simulink model "NE_zad2"  (R2022b)
settings: Solver=ode4  StartTime=0.0  StopTime=1.5  FixedStep=6e-4  RelTol=1e-3
values from neighbouring files (symbols this model uses):
  fie = (UN-IN*Rt)/(wN)    (= 2.67908610996)    [NE_proj_zad2.m]
  IN = 130.7    [NE_proj_zad1_script.m]    (also in NE_proj_zad2.m)
  J = (Js+0*Js)    (= 0.97)    [NE_proj_zad2.m]
  Kp = 1.5*UN/10    (= 66)    [NE_proj_zad1_script.m]    (also in NE_proj_zad2.m)
  KT = 10/(1.2*wN)    (= 0.0548810148593)    [NE_proj_zad1_script.m]    (also in NE_proj_zad2.m)
  Kw = J/(2*KT*kz*beta*fie)    [NE_proj_zad2.m]
  lambdaN = 1.8    [NE_proj_zad1_script.m]    (also in NE_proj_zad2.m)
  m = T1    [NE_proj_zad2.m]
  PN = 54e3    (= 54000)    [NE_proj_zad1_script.m]    (also in NE_proj_zad2.m)
  Rt = 0.254    [NE_proj_zad1_script.m]    (also in NE_proj_zad2.m)
  T = 0.001*Lt/Rt    (= 0.00641732283465)    [NE_proj_zad1_script.m]    (also in NE_proj_zad2.m)
  TR = 4*beta    (= 0.144)    [NE_proj_zad2.m]
  UN = 440    [NE_proj_zad1_script.m]    (also in NE_proj_zad2.m)
  uz0 = lambdaN*IN*(Y*B1)/(B1-beta)    [NE_proj_zad2.m]
  V = beta*(Y*Kp*B)/((B1-beta)*Rt)    [NE_proj_zad2.m]
  wN = nN*pi/30    (= 151.843644924)    [NE_proj_zad1_script.m]    (also in NE_proj_zad2.m)
  Y = 10/(2.5*IN)    (= 0.0306044376435)    [NE_proj_zad1_script.m]    (also in NE_proj_zad2.m = 0.0153022188217)
settings Model: Creator=womru  LastModifiedBy=womru
settings DataIOCC: SaveFormat=StructureWithTime  ReturnWorkspaceOutputs=off
settings OptimizationCC: ReuseModelBlockBuffer=on

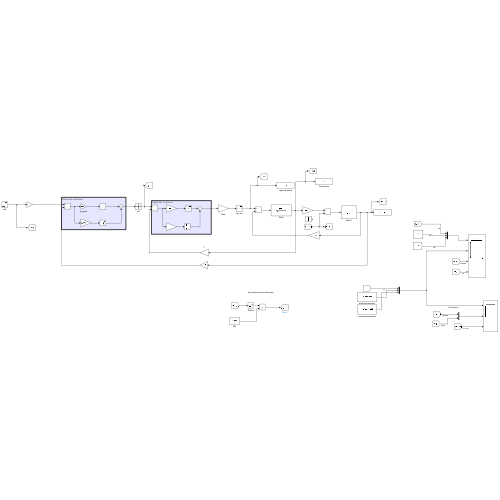
[thumbnail: Simulink's stored preview of the top-level diagram]
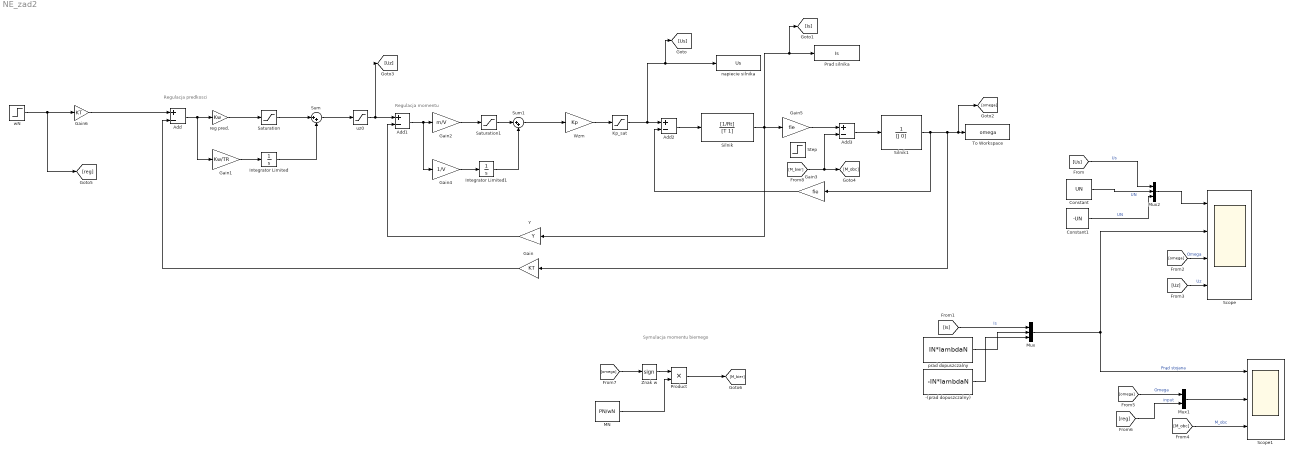
== system NE_zad2 ==
  note: Symulacja momentu biernego
  note: Regulacja momentu
  note: Regulacja predkosci
  -(prad dopuszczalny) : Constant  Value=-IN*lambdaN
  Add{,1..3} (4 alike) : Sum  Inputs=+-
  Constant : Constant  Value=UN
  Constant1 : Constant  Value=-UN
  Gain : Gain  Gain=KT
  Gain1 : Gain  Gain=Kw/TR
  Gain2 : Gain  Gain=m/V
  Gain3 : Gain  Gain=fie
  Gain4 : Gain  Gain=1/V
  Gain5 : Gain  Gain=fie
  Gain6 : Gain  Gain=KT
  Integrator Limited : Integrator  LimitOutput=on  UpperSaturationLimit=10  LowerSaturationLimit=-10
  Integrator Limited1 : Integrator  LimitOutput=on  UpperSaturationLimit=10  LowerSaturationLimit=-10
  Kp_sat : Saturate  UpperLimit=1.5*UN  LowerLimit=-1.5*UN
  MN : Constant  Value=PN/wN
  Mux : Mux  Inputs=3
  Mux1 : Mux  Inputs=2
  Mux2 : Mux  Inputs=3
  Prad silnika : ToWorkspace  VariableName=Is  SaveFormat=Structure With Time  SampleTime=-1
  Product : Product
  Saturation : Saturate  UpperLimit=10  LowerLimit=-10
  Saturation1 : Saturate  UpperLimit=10  LowerLimit=-10
  Scope : Scope  NumInputPorts=4
  Scope1 : Scope  NumInputPorts=3
  Silnik : TransferFcn  Numerator=[1/Rt]  Denominator=[T 1]
  Silnik1 : TransferFcn  Denominator=[J 0]
  Step : Step  Time=0  After=PN/wN  SampleTime=0
  Sum : Sum  Inputs=|++
  Sum1 : Sum  Inputs=|++
  To Workspace : ToWorkspace  VariableName=omega  SaveFormat=Structure With Time  SampleTime=-1
  Wzm : Gain  Gain=Kp
  Y : Gain  Gain=Y
  Znak w : Signum
  napiecie silnika : ToWorkspace  VariableName=Us  SaveFormat=Structure With Time  SampleTime=-1
  prad dopuszczalny : Constant  Value=IN*lambdaN
  reg pred. : Gain  Gain=Kw
  uz0 : Saturate  UpperLimit=abs(uz0)  LowerLimit=-1*abs(uz0)
  wN : Step  Time=0  After=wN  SampleTime=0
  wires:
  Add/1 -> Gain1/1, reg pred./1
  reg pred./1 -> Saturation/1
  Saturation/1 -> Sum/1
  Gain1/1 -> Integrator Limited/1
  Integrator Limited/1 -> Sum/2
  Sum/1 -> uz0/1
  uz0/1 -> [Uz], Add1/1
  Add1/1 -> Gain4/1, Gain2/1
  Gain2/1 -> Saturation1/1
  Saturation1/1 -> Sum1/1
  Sum1/1 -> Wzm/1
  Wzm/1 -> Kp_sat/1
  Gain4/1 -> Integrator Limited1/1
  Integrator Limited1/1 -> Sum1/2
  Add2/1 -> Silnik/1
  Gain5/1 -> Add3/1
  Add3/1 -> Silnik1/1
  Silnik1/1 -> Gain3/1, Gain/1, [omega], To Workspace/1
  Gain3/1 -> Add2/2
  Silnik/1 -> [Is], Prad silnika/1, Y/1, Gain5/1
  Y/1 -> Add1/2
  Gain/1 -> Add/2
  prad dopuszczalny/1 -> Mux/2
  Kp_sat/1 -> [Us], napiecie silnika/1, Add2/1
  [Us] -> Mux2/1  "Us"
  [Is] -> Mux/1  "Is"
  Mux/1 -> Scope1/1, Scope/2  "Prąd stojana"
  [omega] -> Scope/3  "Omega"
  [Uz] -> Scope/4  "Uz"
  Gain6/1 -> Add/1
  [M_obc] -> Scope1/3  "M_obc"
  Mux1/1 -> Scope1/2
  [omega] -> Mux1/1  "Omega"
  [reg] -> Mux1/2  "input"
  -(prad dopuszczalny)/1 -> Mux/3
  wN/1 -> [reg], Gain6/1
  [omega] -> Znak w/1
  Znak w/1 -> Product/1
  Product/1 -> [M_bier]
  MN/1 -> Product/2
  Mux2/1 -> Scope/1
  Constant/1 -> Mux2/2  "UN"
  Constant1/1 -> Mux2/3  "UN"
  [M_bier] -> Add3/2, [M_obc]
